simulink model "Hatch_open_2017b"  (R2020b)
settings: Solver=VariableStepAuto  StartTime=0.0  StopTime=100  RelTol=1e-3
undefined symbols (not defined in the file): sigbuilder_block
libraries: arduinolib x3
settings Model: Creator=shiva  LastModifiedBy=99003727
settings DebuggingCC: SFMachineParentedDataDiag=error  ArithmeticOperatorsInVariantConditions=warning
settings SFSimCC: CustomCodeUndefinedFunction=UseInterfaceOnly

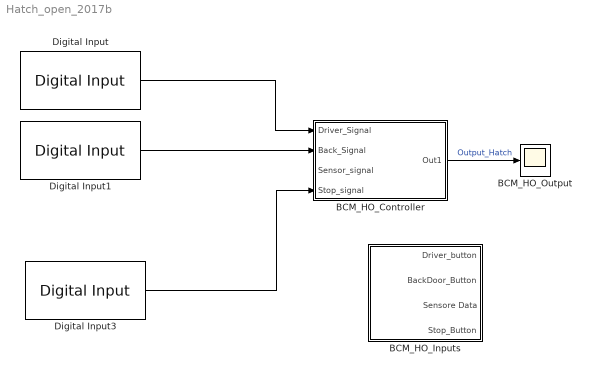
== system Hatch_open_2017b ==
  BCM_HO_Controller : Subsystem
  BCM_HO_Inputs : Subsystem  Tag=STV Subsys  LoadFcn=sigbuilder_block('load');  StartFcn=sigbuilder_block('start');  StopFcn=sigbuilder_block('stop');  ClipboardFcn=sigbuilder_block('clipboard');  mask(Sigbuilder block){tuvar=[0:10]}
      mask help: Simulink:masks:SigbuilderBlock_MD
      mask init:
      | if ~strcmp(get_param(bdroot(gcbh),'SimulationStatus'),'stopped') tuvar = sigbuilder_block('maskInit'); end
      settings: CopyFcn=sigbuilder_block('copy');  DeleteFcn=sigbuilder_block('delete');  ModelCloseFcn=sigbuilder_block('modelClose');  PreSaveFcn=sigbuilder_block('preSave');  PauseFcn=sigbuilder_block('pause');  ContinueFcn=sigbuilder_block('continue');  NameChangeFcn=sigbuilder_block('namechange');  OpenFcn=sigbuilder_block('open',[437.6 199.2 550.4 400 ]);  CloseFcn=sigbuilder_block('close');
      mask Display: plot(0, 0, 100, 100,[2, 2, 32, 32, 2], [68, 8, 8, 68, 68],[32, 2], [38, 38], [32, 19, 2],[53, 60, 44], [32, 17, 17, 2],[16, 16, 31, 31]);txt = getActiveGroup(gcbh);text(2, 100, txt,'verticalAlignment', 'top');
  BCM_HO_Output : Scope
  Digital Input : arduinolib/Digital Input  pinNumber=8  mode=Default  Direction=input  SampleTime=0.1  blockPlatform=arduino
  Digital Input1 : arduinolib/Digital Input  pinNumber=9  mode=Default  Direction=input  SampleTime=0.1  blockPlatform=arduino
  Digital Input3 : arduinolib/Digital Input  pinNumber=10  mode=Default  Direction=input  SampleTime=0.1  blockPlatform=arduino
  wires:
  ? -> BCM_HO_Controller/3(Sensor_signal)  "Sensor_signal"
  BCM_HO_Controller/1(Out1) -> BCM_HO_Output/1  "Output_Hatch"
  Digital Input/1 -> BCM_HO_Controller/1(Driver_Signal)
  Digital Input1/1 -> BCM_HO_Controller/2(Back_Signal)
  Digital Input3/1 -> BCM_HO_Controller/4(Stop_signal)

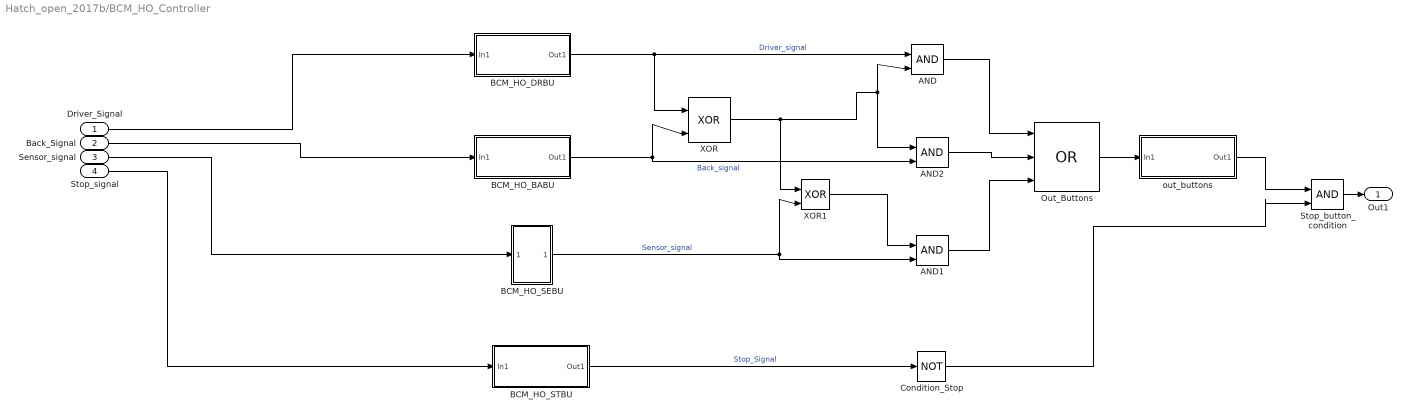
== system Hatch_open_2017b/BCM_HO_Controller ==
  Driver_Signal : Inport
  Back_Signal : Inport  Port=2
  Sensor_signal : Inport  Port=3
  Stop_signal : Inport  Port=4
  AND : Logic  IconShape=distinctive  AllPortsSameDT=off  OutDataTypeStr=boolean
  AND1 : Logic  IconShape=distinctive  AllPortsSameDT=off  OutDataTypeStr=boolean
  AND2 : Logic  IconShape=distinctive  AllPortsSameDT=off  OutDataTypeStr=boolean
  BCM_HO_BABU : Subsystem
  BCM_HO_DRBU : Subsystem
  BCM_HO_SEBU : Subsystem
  BCM_HO_STBU : Subsystem
  Condition_Stop : Logic  Operator=NOT  IconShape=distinctive  AllPortsSameDT=off  OutDataTypeStr=boolean
  Out_Buttons : Logic  Operator=OR  Inputs=3  IconShape=distinctive  AllPortsSameDT=off  OutDataTypeStr=boolean
  Stop_button_condition : Logic  IconShape=distinctive  AllPortsSameDT=off  OutDataTypeStr=boolean
  XOR : Logic  Operator=XOR  IconShape=distinctive  AllPortsSameDT=off  OutDataTypeStr=boolean
  XOR1 : Logic  Operator=XOR  IconShape=distinctive  AllPortsSameDT=off  OutDataTypeStr=boolean
  out_buttons : Subsystem
  Out1 : Outport
  wires:
  BCM_HO_SEBU/1(Out1) -> XOR1/2, AND1/2  "Sensor_signal"
  Stop_signal/1 -> BCM_HO_STBU/1(In1)
  XOR/1 -> XOR1/1, AND2/1, AND/2
  XOR1/1 -> AND1/1
  AND2/1 -> Out_Buttons/2
  Condition_Stop/1 -> Stop_button_condition/2
  BCM_HO_BABU/1(Out1) -> XOR/2, AND2/2  "Back_signal"
  AND/1 -> Out_Buttons/1
  Out_Buttons/1 -> out_buttons/1(In1)
  AND1/1 -> Out_Buttons/3
  BCM_HO_STBU/1(Out1) -> Condition_Stop/1  "Stop_Signal"
  out_buttons/1(Out1) -> Stop_button_condition/1
  BCM_HO_DRBU/1(Out1) -> AND/1, XOR/1  "Driver_signal"
  Sensor_signal/1 -> BCM_HO_SEBU/1(In1)
  Driver_Signal/1 -> BCM_HO_DRBU/1(In1)
  Back_Signal/1 -> BCM_HO_BABU/1(In1)
  Stop_button_condition/1 -> Out1/1

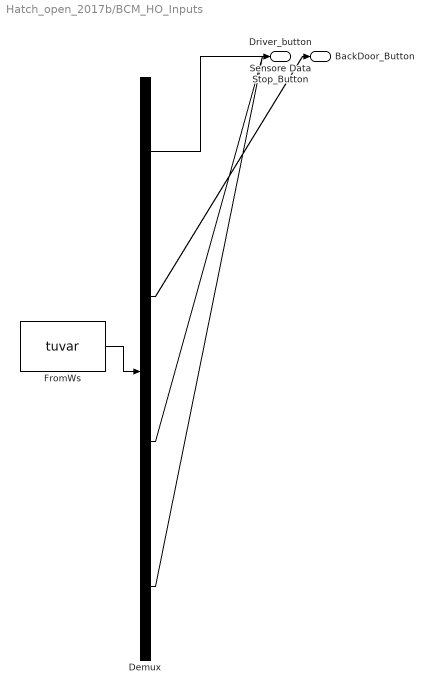
== system Hatch_open_2017b/BCM_HO_Inputs ==
  Demux : Demux  Tag=STV Demux
      settings: DisplayOption=none
  FromWs : FromWorkspace  Tag=STV FromWs  VariableName=tuvar
      SigBuilderData=|
      | common.afterFinalStr = 'Extrapolate'
      | common.sampleTime = 0
      | dataSet.timeRange = [0 100]
      | dataSet.name = 'Group 1'
      | sbobj.Groups.Name = 'Group 1'
      | sbobj.Groups.Signals(1).Name = 'Driver_button'
      | sbobj.Groups.Signals(1).XData = [0 5 5 10 10 15 15 20 20 25 25 30 30 35 35 40 40 45 45 50 50 55 55 60 60 65 65 70 70 75 75 80 80 85 90 95 100]
      | sbobj.Groups.Signals(1).YData = [0 0 1 1 0 0 1 1 0 0 1 1 0 0 1 1 0 0 1 1 0 0 1 1 0 0 1 1 0 0 1 1 0 0 0 0 1]
      | sbobj.Groups.Signals(2).Name = 'BackDoor_Button'
      | sbobj.Groups.Signals(2).XData = [0 5 5 10 10 15 15 20 20 25 25 30 30 35 35 40 40 45 45 50 50 55 55 60 60 65 65 70 70 75 75 80 80 85 85 90 95 100]
      | sbobj.Groups.Signals(2).YData = [1 1 0 0 1 1 0 0 1 1 0 0 1 1 0 0 1 1 0 0 1 1 0 0 1 1 0 0 1 1 0 0 1 1 0 0 0 0]
      | sbobj.Groups.Signals(3).Name = 'Sensore Data'
      | sbobj.Groups.Signals(3).XData = [0 5 10 15 20 25 30 35 40 45 50 55 60 65 70 75 80 85 90 95 100]
      | sbobj.Groups.Signals(3).YData = [2 2 2.5 2.1 3.2 3.5 1.2 0.9 6 2.4 2.9 3.1 2.7 2.8 5 0.9 1.8 2.3 2.7 2.9 3]
      | sbobj.Groups.Signals(4).Name = 'Stop_Button'
      | sbobj.Groups.Signals(4).XData = [0 5 5 10 10 15 15 20 20 25 25 30 30 35 35 40 40 45 45 50 50 55 55 60 60 65 65 70 70 75 80 85 90 95 100]
      | sbobj.Groups.Signals(4).YData = [0 0 1 1 0 0 1 1 0 0 1 1 0 0 1 1 0 0 1 1 0 0 1 1 0 0 1 1 0 0 0 0 0 0 0]
      | sbobj.Groups.TimeRange = [0 100]
  Driver_button : Outport  Tag=STV Outport
  BackDoor_Button : Outport  Tag=STV Outport  Port=2
  Sensore Data : Outport  Tag=STV Outport  Port=3
  Stop_Button : Outport  Tag=STV Outport  Port=4
  wires:
  FromWs/1 -> Demux/1
  Demux/1 -> Driver_button/1
  Demux/2 -> BackDoor_Button/1
  Demux/3 -> Sensore Data/1
  Demux/4 -> Stop_Button/1

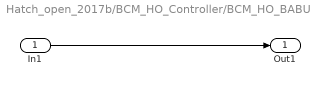
== system Hatch_open_2017b/BCM_HO_Controller/BCM_HO_BABU ==
  In1 : Inport
  Out1 : Outport
  wires:
  In1/1 -> Out1/1

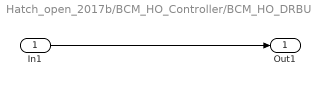
== system Hatch_open_2017b/BCM_HO_Controller/BCM_HO_DRBU ==
  In1 : Inport
  Out1 : Outport
  wires:
  In1/1 -> Out1/1

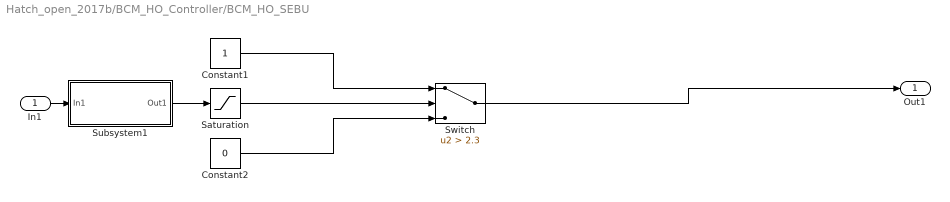
== system Hatch_open_2017b/BCM_HO_Controller/BCM_HO_SEBU ==
  In1 : Inport
  Constant1 : Constant
  Constant2 : Constant  Value=0
  Saturation : Saturate  UpperLimit=3.6  LowerLimit=0
  Subsystem1 : Subsystem
  Switch : Switch  Criteria=u2 > Threshold  Threshold=2.3
  Out1 : Outport
  wires:
  In1/1 -> Subsystem1/1(In1)
  Saturation/1 -> Switch/2
  Constant1/1 -> Switch/1
  Constant2/1 -> Switch/3
  Switch/1 -> Out1/1
  Subsystem1/1(Out1) -> Saturation/1

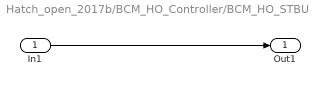
== system Hatch_open_2017b/BCM_HO_Controller/BCM_HO_STBU ==
  In1 : Inport
  Out1 : Outport
  wires:
  In1/1 -> Out1/1

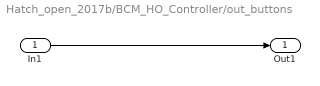
== system Hatch_open_2017b/BCM_HO_Controller/out_buttons ==
  In1 : Inport
  Out1 : Outport
  wires:
  In1/1 -> Out1/1

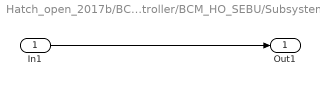
== system Hatch_open_2017b/BCM_HO_Controller/BCM_HO_SEBU/Subsystem1 ==
  In1 : Inport
  Out1 : Outport
  wires:
  In1/1 -> Out1/1
